simulink subsystem "Day1_Scenario_3_4"  (R2024a)
settings: Solver=VariableStepAuto  StartTime=0.0  StopTime=10.0  RelTol=1e-3
libraries: CarMaker4SL x3
settings Model: Creator=junhyung.cha  LastModifiedBy=User

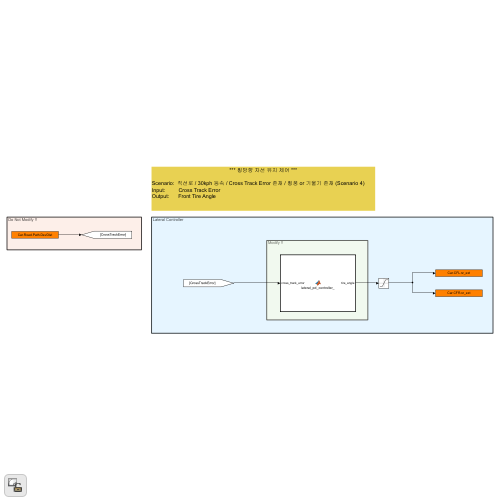
[thumbnail: Simulink's stored preview of the top-level diagram]
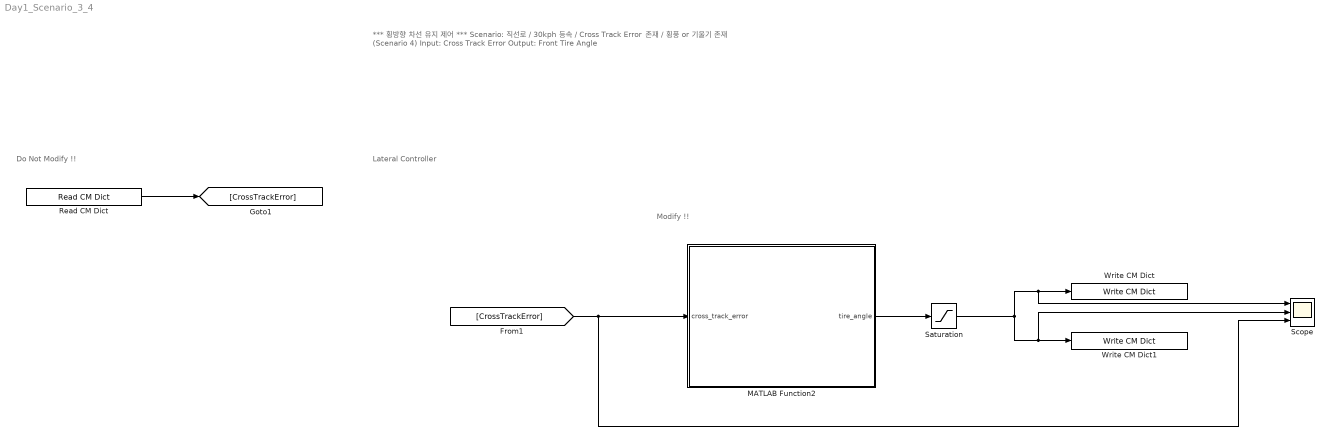
== system Day1_Scenario_3_4 ==
  note: Do Not Modify !!
  note: Modify !!
  note: Lateral Controller
  note: *** 횡방향 차선 유지 제어 ***
      |
      | Scenario: 직선로 / 30kph 등속 / Cross Track Error 존재 / 횡풍 or 기울기 존재 (Scenario 4)
      | Input: Cross Track Error
      | Output: Front Tire Angle
  MATLAB Function2 : MATLAB Function  TreatAsAtomicUnit=on
  Read CM Dict : CarMaker4SL/Read CM Dict  xname=Car.Road.Path.DevDist  xsync=off  xstime=Inherited
  Saturation : Saturate  UpperLimit=2  LowerLimit=-2
  Scope : Scope  NumInputPorts=3
  Write CM Dict : CarMaker4SL/Write CM Dict  xname=Car.CFL.rz_ext  xsync=off
  Write CM Dict1 : CarMaker4SL/Write CM Dict  xname=Car.CFR.rz_ext  xsync=off
  wires:
  Read CM Dict/1 -> [CrossTrackError]
  MATLAB Function2/1(tire_angle) -> Saturation/1
  [CrossTrackError] -> MATLAB Function2/1(cross_track_error), Scope/3
  Saturation/1 -> Write CM Dict/1, Scope/1, Write CM Dict1/1, Scope/2

== matlab function Day1_Scenario_3_4/MATLAB Function2 ==
  settings: updateMethod=DISCRETE  sampleTime=0.05
  data: cross_track_error input; tire_angle output
function tire_angle = lateral_pd_controller_(cross_track_error)
    persistent prev_error Kp Kd step_time initialized
    
    if isempty(initialized)
        Kp = 1.0;        % 비례 이득
        Kd = 1.0;        % 미분 이득
        step_time = 0.001;  % 샘플링 타임
        prev_error = cross_track_error;  % 초기 이전 오차
        initialized = true;
    end
    
    error = cross_track_error;
    derivative = (error - prev_error) / step_time;
    
    tire_angle = - Kp * error - Kd * derivative;
    
    prev_error = error;
end
